simulink model "v2v_urban_scenario_RF_FINAL"  (R2025b)
settings: Solver=FixedStepDiscrete  StartTime=0.0  StopTime=150  RelTol=1e-3
model workspace (MAT data in the model file):
  firstWarning = 1
  originalScenarioChecksum = '39D3C95A58997FFC9DDC4D6B596B4266'
values from neighbouring files (symbols this model uses):
  egoPathS = (0:ds_grid:L)'    [prepare_ego_path.m]
  egoPathX = interp1(s_raw,wp(:,1),egoPathS,'linear')    [prepare_ego_path.m]
  egoPathY = interp1(s_raw,wp(:,2),egoPathS,'linear')    [prepare_ego_path.m]
  RF_ZONE_END_S = 1073.43651801    [rf_scene_calibration.mat]
  RF_ZONE_START_S = 959.172330704    [rf_scene_calibration.mat]
undefined symbols (not defined in the file or in its folder): ADAPTIVE_ENABLE, ATTACK_SEVERITY, CONDITION_CODE, DiscIntNeverNeededParam, RF_TRIGGER, RUN_SEED, SPEED_LIMIT_MPS
libraries: drivingscenarioandsensors x1
settings Model: Creator=Prajwal  LastModifiedBy=Prajwal

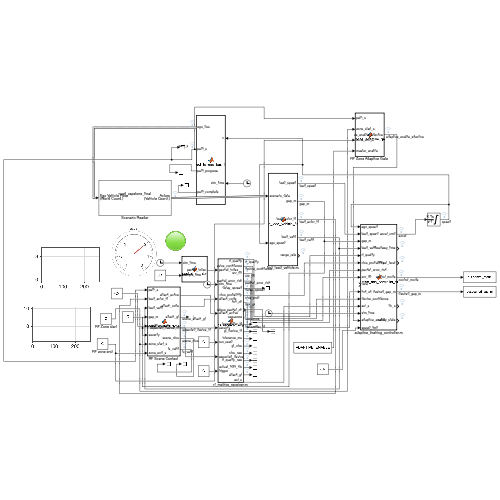
[thumbnail: Simulink's stored preview of the top-level diagram]
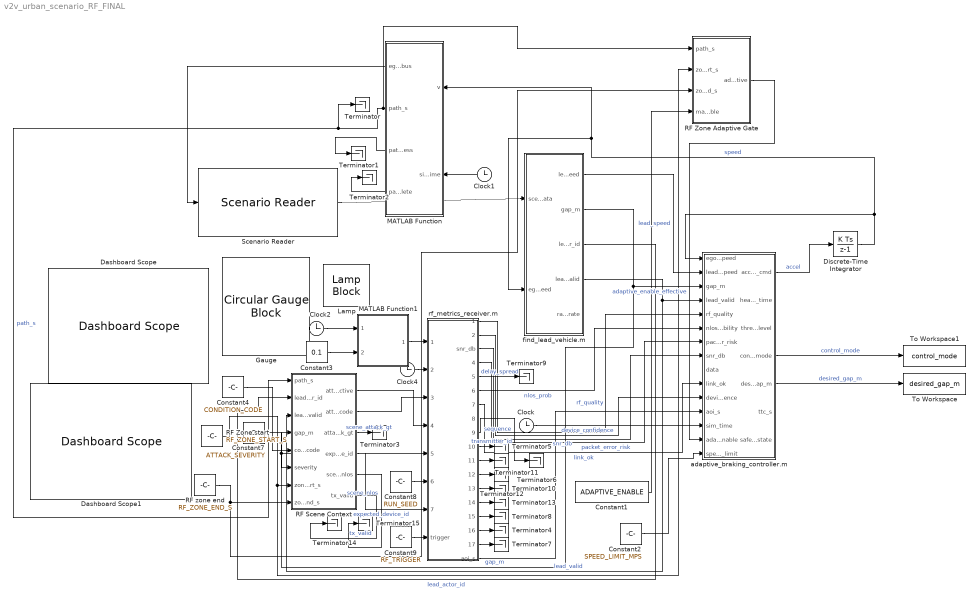
== system v2v_urban_scenario_RF_FINAL ==
  Clock{,1..2,4} (4 alike) : Clock
  Constant1 : Constant  Value=ADAPTIVE_ENABLE  VectorParams1D=off
  Constant2 : Constant  Value=SPEED_LIMIT_MPS
  Constant3 : Constant  Value=0.1
  Constant4 : Constant  Value=CONDITION_CODE
  Constant7 : Constant  Value=ATTACK_SEVERITY
  Constant8 : Constant  Value=RUN_SEED
  Constant9 : Constant  Value=RF_TRIGGER
  Dashboard Scope : DashboardScope  FontColor=[0.0, 0.0, 0.0]
  Dashboard Scope1 : DashboardScope  FontColor=[0.0, 0.0, 0.0]
  Discrete-Time Integrator : DiscreteIntegrator  InitialCondition=8  SampleTime=0.1  LimitOutput=on  UpperSaturationLimit=20  LowerSaturationLimit=0  ICPrevOutput=DiscIntNeverNeededParam  ICPrevScaledInput=DiscIntNeverNeededParam
  Gauge : CircularGaugeBlock  ScaleMin=-4  ScaleMax=2  FontColor=[0.0, 0.0, 0.0]
  Lamp : LampBlock  LabelPosition=Hide  DefaultColor=[192.0, 192.0, 192.0]
  MATLAB Function : MATLAB Function  TreatAsAtomicUnit=on
  MATLAB Function1 : MATLAB Function  TreatAsAtomicUnit=on
  "RF Scene Context " : MATLAB Function  TreatAsAtomicUnit=on
  "RF Zone Adaptive Gate " : MATLAB Function  TreatAsAtomicUnit=on
  RF Zone start : Constant  Value=RF_ZONE_START_S
  RF zone end : Constant  Value=RF_ZONE_END_S
  Scenario Reader : drivingscenarioandsensors/Scenario Reader  ScenarioSource=From file  ScenarioFileName=/Users/Prajwal/Documents/MATLAB/Examples/R2025b/autonomous_control/IntersectionMovementAssistUsingV2VExample3/IntersectionMovementAssist/road_capstone_final.mat  ScenarioVariableName=scenario  OutputCoordinateSystem=Vehicle coordinates  EgoVehicleSource=Input port  EgoVehicleActorID=1  OrientVehiclesOnRoad=off  OutputEgoVehiclePose=off  OutputEgoVehicleState=off  SampleTime=0.1  LaneBoundaryOutput=None  LaneBoundaryDistance=0:0.5:9.5  LaneBoundaryLocation=Center of lane markings  BusNameSource=Auto  BusName=BusActors  BusNumActorsSource=Property  BusNumActors=100  BusName2Source=Auto  BusName2=BusLaneBoundaries  BusNumLaneBoundariesSource=Scenario  BusNumLaneBoundaries=10  BusName3Source=Auto  BusName3=BusEgoActor  BusName4Source=Auto  BusName4=BusEgoState  ShowCoordinateLabels=on  SimulateUsing=Interpreted execution
  Terminator{,1..15} (16 alike) : Terminator
  To Workspace : ToWorkspace  VariableName=desired_gap_m  SaveFormat=Timeseries  SampleTime=-1
  To Workspace1 : ToWorkspace  VariableName=control_mode  SaveFormat=Timeseries  SampleTime=-1
  adaptive_braking_controller.m : MATLAB Function  TreatAsAtomicUnit=on
  find_lead_vehicle.m : MATLAB Function  TreatAsAtomicUnit=on
  rf_metrics_receiver.m : MATLAB Function  TreatAsAtomicUnit=on
  wires:
  Clock/1 -> adaptive_braking_controller.m/13(sim_time)
  find_lead_vehicle.m/1(lead_speed) -> adaptive_braking_controller.m/2(lead_speed)  "lead_speed"
  find_lead_vehicle.m/2(gap_m) -> "RF Scene Context "/4(gap_m), adaptive_braking_controller.m/3(gap_m)  "gap_m"
  rf_metrics_receiver.m/1(rf_quality) -> adaptive_braking_controller.m/5(rf_quality)  "rf_quality"
  rf_metrics_receiver.m/6(nlos_probability) -> adaptive_braking_controller.m/6(nlos_probability)  "nlos_prob"
  rf_metrics_receiver.m/4(packet_error_risk) -> adaptive_braking_controller.m/7(packet_error_risk)  "packet_error_risk"
  adaptive_braking_controller.m/1(accel_cmd) -> Discrete-Time Integrator/1  "accel"
  Discrete-Time Integrator/1 -> adaptive_braking_controller.m/1(ego_speed), MATLAB Function/1(v), find_lead_vehicle.m/2(ego_speed)  "speed"
  rf_metrics_receiver.m/2(device_confidence) -> adaptive_braking_controller.m/11(device_confidence)  "device_confidence"
  Scenario Reader/1 -> find_lead_vehicle.m/1(scenario_data)
  MATLAB Function/1(ego_bus) -> Scenario Reader/1
  adaptive_braking_controller.m/5(desired_gap_m) -> To Workspace/1  "desired_gap_m"
  adaptive_braking_controller.m/4(control_mode) -> To Workspace1/1  "control_mode"
  rf_metrics_receiver.m/3(snr_db) -> adaptive_braking_controller.m/8(snr_db)  "snr_db"
  find_lead_vehicle.m/4(lead_valid) -> "RF Scene Context "/3(lead_valid), adaptive_braking_controller.m/4(lead_valid)  "lead_valid"
  Clock1/1 -> MATLAB Function/2(sim_time)
  rf_metrics_receiver.m/7(link_ok) -> adaptive_braking_controller.m/10(link_ok)  "link_ok"
  rf_metrics_receiver.m/18(aoi_s) -> adaptive_braking_controller.m/12(aoi_s)
  Constant2/1 -> adaptive_braking_controller.m/15(speed_limit)
  Clock2/1 -> MATLAB Function1/1(sim_time)
  Constant3/1 -> MATLAB Function1/2(sample_time)
  MATLAB Function1/1(packet_index) -> rf_metrics_receiver.m/1(packet_index)
  Constant4/1 -> "RF Scene Context "/5(condition_code)
  Constant7/1 -> rf_metrics_receiver.m/5(severity), "RF Scene Context "/6(severity)
  "RF Scene Context "/1(attack_active) -> rf_metrics_receiver.m/4(attack_active)
  "RF Scene Context "/2(attack_code) -> rf_metrics_receiver.m/3(attack_code)
  Clock4/1 -> rf_metrics_receiver.m/2(sim_time)
  Constant8/1 -> rf_metrics_receiver.m/6(run_seed)
  Constant9/1 -> rf_metrics_receiver.m/8(trigger)
  MATLAB Function/2(path_s) -> "RF Zone Adaptive Gate "/1(path_s), "RF Scene Context "/1(path_s), Terminator/1  "path_s"
  MATLAB Function/3(path_progress) -> Terminator1/1
  MATLAB Function/4(path_complete) -> Terminator2/1
  "RF Scene Context "/3(attack_gt) -> Terminator3/1  "scene_attack_gt"
  rf_metrics_receiver.m/5(delay_spread) -> Terminator9/1  "delay_spread"
  rf_metrics_receiver.m/11(gt_device_id) -> Terminator11/1
  rf_metrics_receiver.m/12(inference_ms) -> Terminator12/1
  rf_metrics_receiver.m/13(gt_nlos) -> Terminator10/1
  rf_metrics_receiver.m/14(nlos_raw) -> Terminator13/1
  rf_metrics_receiver.m/15(rf_quality_raw) -> Terminator8/1
  rf_metrics_receiver.m/16(actual_hdf5_idx) -> Terminator4/1
  rf_metrics_receiver.m/17(attack_gt) -> Terminator7/1
  rf_metrics_receiver.m/10(transmitter_id) -> Terminator5/1  "transmitter_id"
  rf_metrics_receiver.m/9(sequence) -> Terminator6/1  "sequence"
  find_lead_vehicle.m/3(lead_actor_id) -> "RF Scene Context "/2(lead_actor_id)  "lead_actor_id"
  RF Zone start/1 -> "RF Zone Adaptive Gate "/2(zone_start_s), "RF Scene Context "/7(zone_start_s)
  RF zone end/1 -> "RF Zone Adaptive Gate "/3(zone_end_s), "RF Scene Context "/8(zone_end_s)
  "RF Scene Context "/4(expected_device_id) -> rf_metrics_receiver.m/7(expected_device_id)  "expected_device_id"
  "RF Scene Context "/5(scene_nlos) -> Terminator15/1  "scene_nlos"
  "RF Scene Context "/6(tx_valid) -> Terminator14/1  "tx_valid"
  Constant1/1 -> "RF Zone Adaptive Gate "/4(master_enable)
  "RF Zone Adaptive Gate "/1(adaptive_enable_effective) -> adaptive_braking_controller.m/14(adaptive_enable)  "adaptive_enable_effective"

== matlab function v2v_urban_scenario_RF_FINAL/MATLAB Function ==
  data: v input; sim_time input; ego_bus output Bus: EgoActorBus; egoPathX parameter; egoPathY parameter; egoPathS parameter; path_s output; path_progress output; path_complete output

function [ego_bus, path_s, path_progress, path_complete] = ...
    speed_to_ego_bus_final(v, sim_time, egoPathX, egoPathY, egoPathS)
%#codegen
%SPEED_TO_EGO_BUS_FINAL Path-locked ego pose with deterministic reset.

TS = 0.1;

persistent sCurrent previousYaw previousTime

if isempty(previousTime)
    sCurrent = 0.0;
    previousYaw = 0.0;
    previousTime = -1.0;
end

if sim_time < previousTime || ...
        (sim_time <= 1.0e-9 && previousTime > 0.0)
    sCurrent = 0.0;
    previousYaw = 0.0;
end
previousTime = sim_time;

pathLength = egoPathS(end);
speed = min(max(double(v),0.0),20.0);
sCurrent = min(sCurrent+speed*TS,pathLength);

x = interp1(egoPathS,egoPathX,sCurrent,'linear');
y = interp1(egoPathS,egoPathY,sCurrent,'linear');

ds = 0.5;
sA = max(sCurrent-ds,0.0);
sB = min(sCurrent+ds,pathLength);

xA = interp1(egoPathS,egoPathX,sA,'linear');
yA = interp1(egoPathS,egoPathY,sA,'linear');
xB = interp1(egoPathS,egoPathX,sB,'linear');
yB = interp1(egoPathS,egoPathY,sB,'linear');

dx = xB-xA;
dy = yB-yA;

if dx == 0.0 && dy == 0.0
    yawDeg = previousYaw;
else
    yawDeg = atan2(dy,dx)*180.0/pi;
end

deltaYaw = yawDeg-previousYaw;
if deltaYaw > 180.0
    deltaYaw = deltaYaw-360.0;
elseif deltaYaw < -180.0
    deltaYaw = deltaYaw+360.0;
end
yawRate = deltaYaw/TS;
previousYaw = yawDeg;

yawRad = yawDeg*pi/180.0;

ego_bus.ActorID = double(9);
ego_bus.Position = [x,y,0.0];
ego_bus.Velocity = [speed*cos(yawRad),speed*sin(yawRad),0.0];
ego_bus.Roll = 0.0;
ego_bus.Pitch = 0.0;
ego_bus.Yaw = yawDeg;
ego_bus.AngularVelocity = [0.0,0.0,yawRate];

path_s = sCurrent;
path_progress = sCurrent/max(pathLength,eps);
path_complete = double(sCurrent >= pathLength-0.25);
end

== matlab function v2v_urban_scenario_RF_FINAL/MATLAB Function1 ==
  data: sim_time input; packet_index output; sample_time input
function packet_index = packet_counter(sim_time, sample_time)
%#codegen
%PACKET_COUNTER Deterministic packet counter reset by simulation time.

Ts = max(double(sample_time),1.0e-3);
packet_index = floor(double(sim_time)/Ts + 1.0e-7);
end

== matlab function v2v_urban_scenario_RF_FINAL/RF Scene Context  ==
  data: path_s input; lead_actor_id input; lead_valid input; gap_m input; attack_active output; condition_code input; severity input; attack_code output; attack_gt output; zone_start_s input; zone_end_s input; expected_device_id output; scene_nlos output; tx_valid output

function [attack_active, attack_code, attack_gt, ...
          expected_device_id, scene_nlos, tx_valid] = ...
    rf_scene_context_dynamic(path_s, lead_actor_id, lead_valid, gap_m, ...
                             condition_code, severity, ...
                             zone_start_s, zone_end_s)
%#codegen
%RF_SCENE_CONTEXT_DYNAMIC
% Scene-conditioned RF experiment logic for the dense second roundabout.
%
% The CURRENT valid lead vehicle is treated as the V2V transmitter.
%
% Inputs:
%   path_s            Ego route position (m)
%   lead_actor_id     Current lead ActorID
%   lead_valid        Current tracker-valid flag
%   gap_m             Current ego-to-lead gap (m)
%   condition_code    0 clean, 1 NLOS, 2 jamming, 3 spoofing
%   severity          Experiment severity in [0,1]
%   zone_start_s      Calibrated RF-zone start path position (m)
%   zone_end_s        Calibrated RF-zone end path position (m)
%
% Outputs:
%   attack_active      RF impairment active flag
%   attack_code        0 outside zone; otherwise selected condition
%   attack_gt          Ground-truth impairment flag for logging only
%   expected_device_id Expected RF device class for current lead
%   scene_nlos         Ground-truth urban-zone flag for logging only
%   tx_valid           A valid V2V transmitting lead is present

MAX_RF_GAP_M = 60.0;
NUM_RF_DEVICE_CLASSES = 3.0;

s0 = min(double(zone_start_s), double(zone_end_s));
s1 = max(double(zone_start_s), double(zone_end_s));

actor_id = floor(double(lead_actor_id));
gap = double(gap_m);

tx_valid_bool = ...
    (double(lead_valid) >= 0.5) && ...
    (actor_id >= 1.0) && ...
    isfinite(gap) && ...
    (gap > 0.0) && ...
    (gap < MAX_RF_GAP_M);

inside_zone = ...
    (double(path_s) >= s0) && ...
    (double(path_s) <= s1);

scene_nlos_bool = tx_valid_bool && inside_zone;

if tx_valid_bool
    expected_device_id = mod(actor_id - 1.0, NUM_RF_DEVICE_CLASSES);
else
    expected_device_id = 0.0;
end

code = floor(double(condition_code));
code = min(max(code,0.0),3.0);

active = ...
    (code > 0.0) && ...
    (double(severity) > 0.0) && ...
    scene_nlos_bool;

tx_valid = double(tx_valid_bool);
scene_nlos = double(scene_nlos_bool);

if active
    attack_active = 1.0;
    attack_code = code;
    attack_gt = 1.0;
else
    attack_active = 0.0;
    attack_code = 0.0;
    attack_gt = 0.0;
end
end

== matlab function v2v_urban_scenario_RF_FINAL/RF Zone Adaptive Gate  ==
  data: path_s input; adaptive_enable_effective output; zone_start_s input; zone_end_s input; master_enable input
function adaptive_enable_effective = rf_zone_adaptive_gate( ...
    path_s, zone_start_s, zone_end_s, master_enable)
%#codegen

z0 = min(double(zone_start_s),double(zone_end_s));
z1 = max(double(zone_start_s),double(zone_end_s));

inside_zone = ...
    double(path_s) >= z0 && ...
    double(path_s) <= z1;

adaptive_enable_effective = double( ...
    double(master_enable) >= 0.5 && inside_zone);
end

== matlab function v2v_urban_scenario_RF_FINAL/adaptive_braking_controller.m ==
  data: ego_speed input; accel_cmd output; lead_speed input; gap_m input; lead_valid input; rf_quality input; nlos_probability input; packet_error_risk input; snr_db input; data input; headway_time output; threat_level output; link_ok input; device_confidence input; aoi_s input; sim_time input; control_mode output; desired_gap_m output; adaptive_enable input; speed_limit input; ttc_s output; safety_state output

function [accel_cmd, headway_time, threat_level, control_mode, ...
          desired_gap_m, ttc_s, safety_state] = ...
    adaptive_acc_controller_final( ...
    ego_speed, lead_speed, gap_m, lead_valid, rf_quality, ...
    nlos_probability, packet_error_risk, snr_db, data, link_ok, ...
    device_confidence, aoi_s, sim_time, adaptive_enable, speed_limit)
%#codegen
% Fixed or RF-adaptive IDM-based ACC.

TS = 0.1;
MIN_STANDSTILL_GAP_M = 2.5;
HEADWAY_NOMINAL_S = 1.5;
HEADWAY_MAX_S = 2.8;
HEADWAY_FILTER_TAU_S = 0.6;
FREE_ACCEL_MPS2 = 1.4;
COMFORT_DECEL_MAG_MPS2 = 2.5;
IDM_EXPONENT = 4.0;
MAX_ACCEL_MPS2 = 1.5;
MAX_SERVICE_DECEL_MPS2 = -4.0;
MAX_EMERGENCY_DECEL_MPS2 = -7.5;
NORMAL_BRAKE_JERK_MPS3 = -3.0;
EMERGENCY_BRAKE_JERK_MPS3 = -15.0;
ACCEL_JERK_MPS3 = 2.0;

persistent headway_state accel_state previous_time

if isempty(previous_time)
    headway_state = HEADWAY_NOMINAL_S;
    accel_state = 0.0;
    previous_time = -1.0;
end

if sim_time < previous_time || ...
        (sim_time <= 1.0e-9 && previous_time > 0.0)
    headway_state = HEADWAY_NOMINAL_S;
    accel_state = 0.0;
end
previous_time = sim_time;

v = max(double(ego_speed),0.0);
vLead = max(double(lead_speed),0.0);
vSet = min(max(double(speed_limit),3.0),20.0);
hasLead = lead_valid >= 0.5;

q = min(max(double(rf_quality),0.0),1.0);
pn = min(max(double(nlos_probability),0.0),1.0);
per = min(max(double(packet_error_risk),0.0),1.0);
conf = min(max(double(device_confidence),0.0),1.0);
staleRisk = min(max(double(aoi_s),0.0),1.0);

if adaptive_enable >= 0.5
    risk = 0.45*(1.0-q) + 0.20*pn + 0.15*per + ...
           0.10*(1.0-conf) + 0.10*staleRisk;
    if link_ok < 0.5
        risk = 1.0;
    elseif conf < 0.35
        % Wrong or weak RF fingerprint: retain radar authority but command a
        % conservative time-gap policy.
        risk = max(risk,0.85);
    end
    risk = min(max(risk,0.0),1.0);
    commandedHeadway = HEADWAY_NOMINAL_S + ...
        (HEADWAY_MAX_S-HEADWAY_NOMINAL_S)*risk;
else
    risk = 0.0;
    commandedHeadway = HEADWAY_NOMINAL_S;
end

alpha = TS/(HEADWAY_FILTER_TAU_S+TS);
headway_state = headway_state + alpha*(commandedHeadway-headway_state);
headway_state = min(max(headway_state,HEADWAY_NOMINAL_S),HEADWAY_MAX_S);
headway_time = headway_state;

desired_gap_m = MIN_STANDSTILL_GAP_M+headway_time*v;

speedRatio = v/max(vSet,0.1);
aDesired = FREE_ACCEL_MPS2*(1.0-speedRatio^IDM_EXPONENT);

closingSpeed = 0.0;
ttc_s = 1.0e6;

if hasLead
    gap = max(double(gap_m),0.10);
    closingSpeed = v-vLead;

    if closingSpeed > 0.10
        ttc_s = gap/closingSpeed;
    end

    dynamicTerm = v*closingSpeed / ...
        (2.0*sqrt(FREE_ACCEL_MPS2*COMFORT_DECEL_MAG_MPS2));
    dynamicDesiredGap = MIN_STANDSTILL_GAP_M + ...
        max(0.0,v*headway_time+dynamicTerm);

    aDesired = FREE_ACCEL_MPS2 * ...
        (1.0-speedRatio^IDM_EXPONENT-(dynamicDesiredGap/gap)^2);
end

aDesired = min(max(aDesired,MAX_SERVICE_DECEL_MPS2),MAX_ACCEL_MPS2);

safety_state = 0.0;

if hasLead
    gap = max(double(gap_m),0.0);
    availableGap = max(gap-MIN_STANDSTILL_GAP_M,0.25);

    if gap <= 0.05
        safety_state = 3.0;
        aDesired = MAX_EMERGENCY_DECEL_MPS2;
    elseif ttc_s < 0.75 || gap < 0.75
        safety_state = 2.0;
        aDesired = MAX_EMERGENCY_DECEL_MPS2;
    elseif closingSpeed > 0.10
        requiredDecel = -(closingSpeed^2)/(2.0*availableGap);
        if ttc_s < 1.8 || requiredDecel < MAX_SERVICE_DECEL_MPS2
            safety_state = 2.0;
            aDesired = min(aDesired,max(requiredDecel,MAX_EMERGENCY_DECEL_MPS2));
        elseif ttc_s < 3.0
            safety_state = 1.0;
        end
    end
end

if safety_state >= 2.0
    lowerStep = accel_state+EMERGENCY_BRAKE_JERK_MPS3*TS;
else
    lowerStep = accel_state+NORMAL_BRAKE_JERK_MPS3*TS;
end
upperStep = accel_state+ACCEL_JERK_MPS3*TS;

accel_cmd = min(max(aDesired,lowerStep),upperStep);
if safety_state == 3.0
    accel_cmd = MAX_EMERGENCY_DECEL_MPS2;
end
accel_cmd = min(max(accel_cmd,MAX_EMERGENCY_DECEL_MPS2),MAX_ACCEL_MPS2);
accel_state = accel_cmd;

if safety_state >= 2.0
    control_mode = 4.0;
elseif adaptive_enable >= 0.5 && (link_ok < 0.5 || conf < 0.35)
    control_mode = 3.0;
elseif adaptive_enable >= 0.5 && hasLead && risk > 0.25
    control_mode = 2.0;
elseif hasLead
    control_mode = 1.0;
else
    control_mode = 0.0;
end

if safety_state >= 2.0
    threat_level = 4.0;
elseif adaptive_enable >= 0.5 && (link_ok < 0.5 || conf < 0.25)
    threat_level = 3.0;
elseif adaptive_enable >= 0.5 && ...
       (pn > 0.60 || q < 0.40 || snr_db < 5.0)
    threat_level = 2.0;
elseif adaptive_enable >= 0.5 && risk > 0.25
    threat_level = 1.0;
else
    threat_level = 0.0;
end
end

== matlab function v2v_urban_scenario_RF_FINAL/rf_metrics_receiver.m ==
  data: packet_index input; sim_time input; attack_code input; attack_active input; severity input; run_seed input; expected_device_id input; rf_quality output; trigger input; device_confidence output; snr_db output; packet_error_risk output; delay_spread output; nlos_probability output; link_ok output; wireless_packet_ok output; sequence output; transmitter_id output; gt_device_id output; inference_ms output; gt_nlos output; nlos_raw output; rf_quality_raw output; actual_hdf5_idx output; attack_gt output; aoi_s output

function [rf_quality, device_confidence, snr_db, packet_error_risk, ...
          delay_spread, nlos_probability, link_ok, wireless_packet_ok, ...
          sequence, transmitter_id, gt_device_id, inference_ms, gt_nlos, ...
          nlos_raw, rf_quality_raw, actual_hdf5_idx, attack_gt, aoi_s] = ...
    rf_metrics_receiver_experiment( ...
          packet_index, sim_time, attack_code, attack_active, severity, ...
          run_seed, expected_device_id, trigger)
%#codegen
%RF_METRICS_RECEIVER_EXPERIMENT Separate SIL health from wireless delivery.
%
% link_ok:
%   Valid localhost MATLAB/Python transaction.
%
% wireless_packet_ok:
%   Simulated V2V delivery result generated from the channel/PER model.
%
% The raw CNN outputs are always logged on a valid SIL response. Controller
% metrics update only when the simulated wireless packet is delivered.

coder.extrinsic('v2v_zmq_request_experiment');
coder.extrinsic('decode_v2v_json_experiment');

persistent haveDelivered lastQ lastConf lastSNR lastPER lastDS lastNLOS
persistent lastServerSequence lastDeliveredTime previousPacketIndex

if isempty(previousPacketIndex)
    haveDelivered = false;
    lastQ = 0.25;
    lastConf = 0.0;
    lastSNR = -5.0;
    lastPER = 1.0;
    lastDS = 1.0e-6;
    lastNLOS = 0.5;
    lastServerSequence = -1.0;
    lastDeliveredTime = double(sim_time);
    previousPacketIndex = -1.0;
end

if double(packet_index) < previousPacketIndex
    haveDelivered = false;
    lastServerSequence = -1.0;
    lastDeliveredTime = double(sim_time);
end
previousPacketIndex = double(packet_index);

% Conservative finite defaults.
rf_quality = 0.25;
device_confidence = 0.0;
snr_db = -5.0;
packet_error_risk = 1.0;
delay_spread = 1.0e-6;
nlos_probability = 0.5;
link_ok = 0.0;
wireless_packet_ok = 0.0;
sequence = lastServerSequence;
transmitter_id = -1.0;
gt_device_id = -1.0;
inference_ms = 0.0;
gt_nlos = 0.0;
nlos_raw = 0.5;
rf_quality_raw = 0.25;
actual_hdf5_idx = -1.0;
attack_gt = double(attack_active >= 0.5);
aoi_s = max(double(sim_time)-lastDeliveredTime,0.0);

if trigger < 0.5
    return;
end

raw = repmat(' ',1,0);
coder.varsize('raw',[1 4096],[0 1]);

raw = v2v_zmq_request_experiment(packet_index,sim_time, ...
    attack_code,attack_active,severity,run_seed,expected_device_id);

if isempty(raw)
    if haveDelivered
        rf_quality = min(lastQ,0.35);
        device_confidence = min(lastConf,0.25);
        snr_db = lastSNR;
        packet_error_risk = max(lastPER,0.80);
        delay_spread = lastDS;
        nlos_probability = lastNLOS;
    end
    return;
end

values = zeros(1,19);
values = decode_v2v_json_experiment(raw);

if values(1) < 0.5
    return;
end

newSequence = values(8);
if lastServerSequence >= 0.0 && newSequence <= lastServerSequence
    return;
end

link_ok = 1.0;
lastServerSequence = newSequence;
sequence = newSequence;

rf_quality_raw = values(2);
nlos_raw = values(7);
transmitter_id = values(9);
gt_device_id = values(10);
inference_ms = values(11);
gt_nlos = values(12);
wireless_packet_ok = values(13);
actual_hdf5_idx = values(14);
attack_gt = values(16);

if wireless_packet_ok >= 0.5
    rf_quality = values(2);

    % Convert raw classifier confidence into identity trust. A highly
    % confident prediction for the wrong transmitter must not be treated as
    % trusted V2V identity.
    predicted_id = values(9);
    expected_id = values(18);
    if round(predicted_id) == round(expected_id)
        device_confidence = values(3);
    else
        device_confidence = 0.0;
    end

    snr_db = values(4);
    packet_error_risk = values(5);
    delay_spread = values(6);
    nlos_probability = values(7);

    lastQ = rf_quality;
    lastConf = device_confidence;
    lastSNR = snr_db;
    lastPER = packet_error_risk;
    lastDS = delay_spread;
    lastNLOS = nlos_probability;
    lastDeliveredTime = double(sim_time);
    haveDelivered = true;
elseif haveDelivered
    rf_quality = lastQ;
    device_confidence = lastConf;
    snr_db = lastSNR;
    packet_error_risk = lastPER;
    delay_spread = lastDS;
    nlos_probability = lastNLOS;
end

aoi_s = max(double(sim_time)-lastDeliveredTime,0.0);
end

== matlab function v2v_urban_scenario_RF_FINAL/find_lead_vehicle.m ==
  data: lead_speed output; gap_m output; lead_actor_id output; scenario_data input; ego_speed input; lead_valid output; range_rate output

function [lead_speed, gap_m, lead_actor_id, lead_valid, range_rate] = ...
    find_lead_vehicle_final(scenario_data, ego_speed)
%#codegen
% Generic nearest in-lane lead tracker for Scenario Reader VEHICLE coordinates.

TS = 0.1;
MAX_LOOK_AHEAD_M = 100.0;
MIN_FORWARD_ORIGIN_M = 1.0;
BASE_LATERAL_GATE_M = 1.9;
LATERAL_GATE_SLOPE = 0.020;
MAX_LATERAL_GATE_M = 3.5;
MAX_NEW_TARGET_YAW_DEG = 50.0;
MAX_LOCKED_TARGET_YAW_DEG = 70.0;
PERSISTENCE_SAMPLES = 3.0;
LOSS_GRACE_SAMPLES = 3.0;
SWITCH_ADVANTAGE_M = 1.0;
ORIGIN_TO_BUMPER_M = 4.2;
RANGE_RATE_ALPHA = 0.35;
MAX_ABS_RANGE_RATE_MPS = 40.0;

persistent locked_id locked_lon locked_speed
persistent pending_id pending_count lost_count
persistent previous_lon filtered_range_rate had_range previous_time

sim_time = double(scenario_data.Time);

if isempty(previous_time)
    locked_id = -1.0;
    locked_lon = MAX_LOOK_AHEAD_M + ORIGIN_TO_BUMPER_M;
    locked_speed = max(double(ego_speed),0.0);
    pending_id = -1.0;
    pending_count = 0.0;
    lost_count = 0.0;
    previous_lon = 0.0;
    filtered_range_rate = 0.0;
    had_range = false;
    previous_time = -1.0;
end

if sim_time < previous_time || ...
        (sim_time <= 1.0e-9 && previous_time > 0.0)
    locked_id = -1.0;
    locked_lon = MAX_LOOK_AHEAD_M + ORIGIN_TO_BUMPER_M;
    locked_speed = max(double(ego_speed),0.0);
    pending_id = -1.0;
    pending_count = 0.0;
    lost_count = 0.0;
    previous_lon = 0.0;
    filtered_range_rate = 0.0;
    had_range = false;
end
previous_time = sim_time;

actors = scenario_data.Actors;
n = min(int32(double(scenario_data.NumActors)),int32(numel(actors)));

raw_id = -1.0;
raw_lon = MAX_LOOK_AHEAD_M + ORIGIN_TO_BUMPER_M;
raw_speed = max(double(ego_speed),0.0);

locked_visible = false;
locked_lon_now = locked_lon;
locked_speed_now = locked_speed;

for i = 1:n
    actor_id = double(actors(i).ActorID);
    if actor_id <= 0.0
        continue;
    end

    lon = double(actors(i).Position(1));
    lat = double(actors(i).Position(2));
    relative_yaw = mod(double(actors(i).Yaw)+180.0,360.0)-180.0;

    lateral_gate = min(MAX_LATERAL_GATE_M, ...
        BASE_LATERAL_GATE_M + LATERAL_GATE_SLOPE*max(lon,0.0));

    actor_speed = hypot(double(actors(i).Velocity(1)), ...
                        double(actors(i).Velocity(2)));

    new_valid = lon > MIN_FORWARD_ORIGIN_M && ...
        lon < MAX_LOOK_AHEAD_M + ORIGIN_TO_BUMPER_M && ...
        abs(lat) < lateral_gate && ...
        abs(relative_yaw) < MAX_NEW_TARGET_YAW_DEG;

    if actor_id == locked_id
        locked_valid = lon > 0.0 && ...
            lon < MAX_LOOK_AHEAD_M + ORIGIN_TO_BUMPER_M + 6.0 && ...
            abs(lat) < lateral_gate + 0.8 && ...
            abs(relative_yaw) < MAX_LOCKED_TARGET_YAW_DEG;

        if locked_valid
            locked_visible = true;
            locked_lon_now = lon;
            locked_speed_now = actor_speed;
        end
    end

    if new_valid && lon < raw_lon
        raw_id = actor_id;
        raw_lon = lon;
        raw_speed = actor_speed;
    end
end

if locked_id < 0.0
    if raw_id >= 0.0
        locked_id = raw_id;
        locked_lon = raw_lon;
        locked_speed = raw_speed;
    end
    pending_id = -1.0;
    pending_count = 0.0;
    lost_count = 0.0;

elseif locked_visible
    locked_lon = locked_lon_now;
    locked_speed = locked_speed_now;
    lost_count = 0.0;

    if raw_id == locked_id || raw_id < 0.0
        pending_id = -1.0;
        pending_count = 0.0;
    elseif raw_lon < locked_lon_now-SWITCH_ADVANTAGE_M
        if pending_id == raw_id
            pending_count = pending_count+1.0;
        else
            pending_id = raw_id;
            pending_count = 1.0;
        end

        if pending_count >= PERSISTENCE_SAMPLES
            locked_id = raw_id;
            locked_lon = raw_lon;
            locked_speed = raw_speed;
            pending_id = -1.0;
            pending_count = 0.0;
            had_range = false;
        end
    else
        pending_id = -1.0;
        pending_count = 0.0;
    end
else
    lost_count = lost_count+1.0;

    if raw_id >= 0.0
        if pending_id == raw_id
            pending_count = pending_count+1.0;
        else
            pending_id = raw_id;
            pending_count = 1.0;
        end

        if pending_count >= PERSISTENCE_SAMPLES
            locked_id = raw_id;
            locked_lon = raw_lon;
            locked_speed = raw_speed;
            pending_id = -1.0;
            pending_count = 0.0;
            lost_count = 0.0;
            had_range = false;
        end
    elseif lost_count >= LOSS_GRACE_SAMPLES
        locked_id = -1.0;
        locked_lon = MAX_LOOK_AHEAD_M + ORIGIN_TO_BUMPER_M;
        locked_speed = max(double(ego_speed),0.0);
        pending_id = -1.0;
        pending_count = 0.0;
        lost_count = 0.0;
        had_range = false;
    end
end

if locked_id >= 0.0
    lead_actor_id = locked_id;
    lead_valid = 1.0;
    gap_m = max(locked_lon-ORIGIN_TO_BUMPER_M,0.0);

    if had_range
        raw_rate = (locked_lon-previous_lon)/TS;
        raw_rate = min(max(raw_rate,-MAX_ABS_RANGE_RATE_MPS), ...
                       MAX_ABS_RANGE_RATE_MPS);
        filtered_range_rate = filtered_range_rate + ...
            RANGE_RATE_ALPHA*(raw_rate-filtered_range_rate);
    else
        filtered_range_rate = locked_speed-max(double(ego_speed),0.0);
    end

    previous_lon = locked_lon;
    had_range = true;
    range_rate = filtered_range_rate;

    speed_from_range = max(double(ego_speed)+range_rate,0.0);
    if abs(locked_speed-speed_from_range) <= 4.0
        lead_speed = 0.65*locked_speed+0.35*speed_from_range;
    else
        lead_speed = speed_from_range;
    end
else
    lead_speed = max(double(ego_speed),0.0);
    gap_m = MAX_LOOK_AHEAD_M;
    lead_actor_id = -1.0;
    lead_valid = 0.0;
    range_rate = 0.0;
    had_range = false;
end
end
